simulink model "sched"  (R2020b)
settings: Solver=ode45  StartTime=0.0  StopTime=4.8  RelTol=1e-3  EnableMultiTasking=on
InitFcn:
  | clear functions
libraries: truetime x1
settings Model: ExtModeTrigMode=oneshot  ExtModeArmWhenConnect=off  ExtModeAutoUpdateStatusClock=off  Creator=anton  LastModifiedBy=sunandan
settings DataIOCC: SaveFormat=Array  SignalLoggingSaveFormat=ModelDataLogs  ReturnWorkspaceOutputs=off
settings OptimizationCC: BlockReduction=off  BooleanDataType=off  ExpressionDepthLimit=2147483647  LifeSpan=inf
settings DebuggingCC: SaveWithParameterizedLinksMsg=none  UnderspecifiedInitializationDetection=Classic  MergeDetectMultiDrivingBlocksExec=none  SignalResolutionControl=TryResolveAllWithWarning  MultiTaskDSMMsg=warning  MultiTaskCondExecSysMsg=none  FcnCallInpInsideContextMsg=warning  StateNameClashWarn=warning  SFUnexpectedBacktrackingDiag=warning  SFNoUnconditionalDefaultTransitionDiag=warning  SFExecutionAtInitializationDiag=none  ArithmeticOperatorsInVariantConditions=warning
settings HardwareCC: ProdBitPerPointer=32  ProdBitPerSizeT=32  ProdBitPerPtrDiffT=32  ProdLargestAtomicFloat=None  ProdIntDivRoundTo=Undefined  ProdEndianess=Unspecified  ProdWordSize=32  ProdHWDeviceType=32-bit Generic  TargetUnknown=on
settings ModelReferenceCC: PropagateSignalLabelsOutOfModel=off
settings SFSimCC: SimUseLocalCustomCode=off  CustomCodeUndefinedFunction=UseInterfaceOnly
settings RTWCC: RTWUseLocalCustomCode=off
settings CodeAppCC: StateflowObjectComments=on
settings GRTTargetCC: TargetLangStandard=C89/C90 (ANSI)  CombineOutputUpdateFcns=off  GRTInterface=on
settings ConfigComp: CovMetricSettings=dw  CovSaveCumulativeToWorkspaceVar=on  CovSaveSingleToWorkspaceVar=on  CovExternalEMLEnable=off

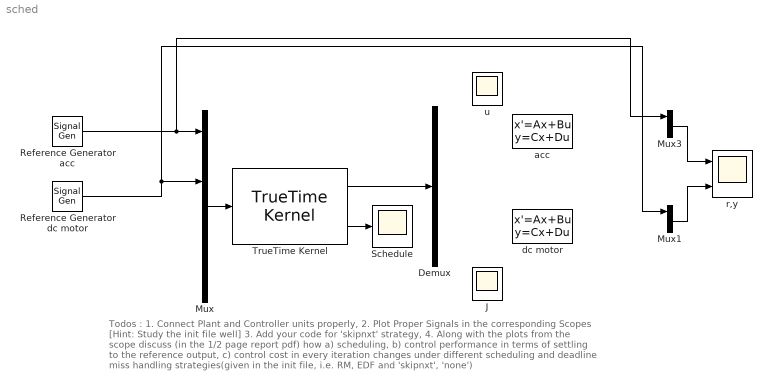
== system sched ==
  note: Todos :
      | 1. Connect Plant and Controller units properly,
      | 2. Plot Proper Signals in the corresponding Scopes
      | [Hint: Study the init file well]
      | 3. Add your code for 'skipnxt' strategy,
      | 4. Along with the plots from the scope discuss (in the 1/2 page report pdf) how
      | a) scheduling,
      | b) control performance in terms of settling to the reference output,
      | c) control cost in every iteration
      | changes under different scheduling and deadline miss handling strategies(given in the init file, i.e. RM, EDF and 'skipnxt', 'none')
  Demux : Demux
      settings: DisplayOption=none
  J : Scope  NumInputPorts=2
  Mux : Mux
  Mux1 : Mux  Inputs=2
  Mux3 : Mux  Inputs=2
  Reference Generator acc : SignalGenerator  WaveForm=square  Amplitude=-10  Frequency=0.02
  Reference Generator dc motor : SignalGenerator  WaveForm=square  Amplitude=-1  Frequency=0.02
  Schedule : Scope
  TrueTime Kernel : truetime/TrueTime Kernel  sfun=sched_init  args=12  ninputsoutputs=[4 4]  ntriggers=0  trigtype=falling  nwnodenbr=[]  clockoffsetdrift=[0 0]  schedoutput=on  battery=off  poweroutput=off
  acc : StateSpace  A=[0 1; 1 0]  B=[0; 1]  C=[1 0]  D=[0]  InitialCondition=[0;0]
  dc motor : StateSpace  A="[-0.9999    0.9998; -0.0200   -1.9998]"  B=[0.0002;1.9999]  C=[1 0]  D=[0]  InitialCondition=[0;0]
  r,y : Scope  NumInputPorts=2
  u : Scope  NumInputPorts=2
  wires:
  Mux/1 -> TrueTime Kernel/1
  TrueTime Kernel/1 -> Demux/1
  Mux1/1 -> r,y/2
  Mux3/1 -> r,y/1
  TrueTime Kernel/2 -> Schedule/1
  Reference Generator dc motor/1 -> Mux/2, Mux1/1
  Reference Generator acc/1 -> Mux3/1, Mux/1
